simulink model "mpc_doubleint"  (Simulink 7.0)
settings: Solver=ode45  SolverMode=SingleTasking  StartTime=0.0  StopTime=5  RelTol=1e-3
values from neighbouring files (symbols this model uses):
  r = 1    [mpcdoubleint.m]    (also in mpcmiso.m; mpcmotor.m = pi*ones(Tf,2); mpcoffsets.m = r0*ones(Tf,1); mpcpreview.m = [ones(5,1);0.5*ones(p-5,1)])
  x01 = 0    [mpcdoubleint.m]
  x02 = 0    [mpcdoubleint.m]
libraries: mpclib x1
settings Model: Creator=rchen  LastModifiedBy=rchen  ExtModeTrigMode=oneshot  ExtModeArmWhenConnect=off
settings DataIOCC: LimitDataPoints=off  SignalLoggingName=sigsOut
settings OptimizationCC: BooleanDataType=off  InlineInvariantSignals=on
settings DebuggingCC: SaveWithParameterizedLinksMsg=none  SignalResolutionControl=TryResolveAllWithWarning  SolverPrmCheckMsg=none  MultiTaskDSMMsg=warning  MultiTaskCondExecSysMsg=none  IntegerOverflowMsg=none  StrictBusMsg=None
settings HardwareCC: TargetUnknown=on
settings RTWCC: IncludeERTFirstTime=on
settings GRTTargetCC: TargetFcnLib=ansi_tfl_tmw.mat

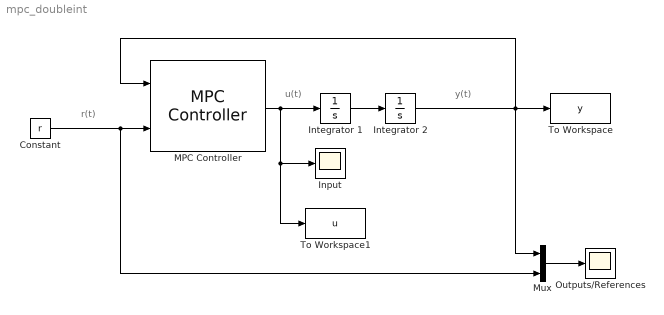
== system mpc_doubleint ==
  note: u(t)
  note: y(t)
  note: r(t)
  Constant : Constant  Value=r  OutDataType=sfix(16)  OutScaling=2^0
  Input : Scope
      settings: TimeRange=6  YMin=-1  YMax=1  DataFormat=Structure
  Integrator 1 : Integrator  InitialCondition=x01  UpperSaturationLimit=Inf  LowerSaturationLimit=-Inf
  Integrator 2 : Integrator  InitialCondition=x02  UpperSaturationLimit=Inf  LowerSaturationLimit=-Inf
  MPC Controller : mpclib/MPC Controller  SystemSampleTime=-1  mpcobj=mpc_controller  n_mv=0  x0=[]  ref_from_ws=off  ref_signal_name=[]  ref_preview=on  md_from_ws=off  md_signal_name=[]  md_preview=on  from_project=off  md_inport=off  mv_inport=off  lims_inport=off  project_file=MPCtask.mat
  Mux : Mux  Inputs=2
  Outputs/References : Scope
      settings: TimeRange=5  YMin=0  YMax=1.5  DataFormat=Structure
  To Workspace : ToWorkspace  VariableName=y  SampleTime=-1  SaveFormat=Array
      settings: MaxDataPoints=Inf
  To Workspace1 : ToWorkspace  VariableName=u  SampleTime=-1  SaveFormat=Array
      settings: MaxDataPoints=Inf
  wires:
  MPC Controller/1 -> Integrator 1/1, Input/1, To Workspace1/1
  Integrator 2/1 -> To Workspace/1, Mux/1, MPC Controller/1
  Mux/1 -> Outputs/References/1
  Constant/1 -> MPC Controller/2, Mux/2
  Integrator 1/1 -> Integrator 2/1
